simulink model "florianMaierSimulink"  (R2021b)
settings: Solver=VariableStepAuto  StartTime=0.0  StopTime=360*16*365  RelTol=1e-3
settings Model: Creator=philippsum  LastModifiedBy=philippsum

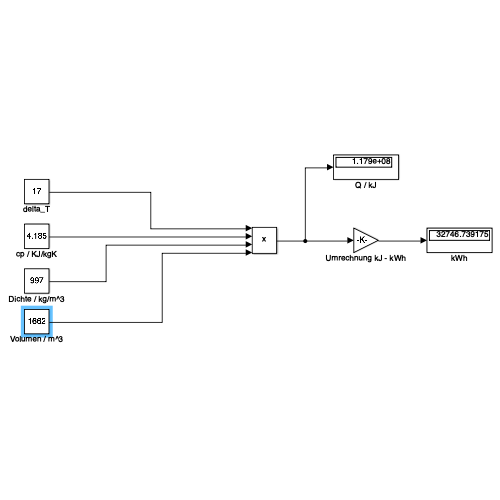
[thumbnail: Simulink's stored preview of the top-level diagram]
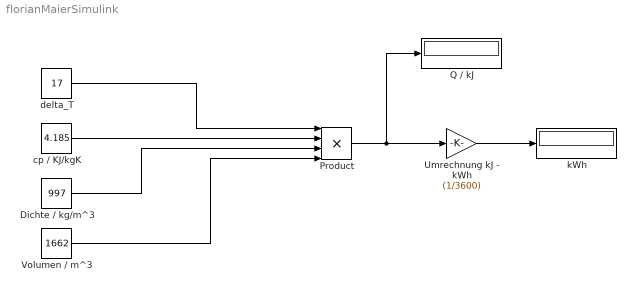
== system florianMaierSimulink ==
  Dichte / kg/m^3 : Constant  Value=997
  Product : Product  Inputs=4
  Q / kJ : Display
  Umrechnung kJ - kWh : Gain  Gain=(1/3600)
  Volumen / m^3 : Constant  Value=1662
  cp / KJ/kgK : Constant  Value=4.185
  delta_T : Constant  Value=17
  kWh : Display
  wires:
  delta_T/1 -> Product/1
  cp / KJ/kgK/1 -> Product/2
  Dichte / kg/m^3/1 -> Product/3
  Volumen / m^3/1 -> Product/4
  Product/1 -> Umrechnung kJ - kWh/1, Q / kJ/1
  Umrechnung kJ - kWh/1 -> kWh/1
